simulink library "csu_elk_est_landed_kinematics_lib"  (R2015b)
settings: Solver=ode45  StartTime=0.0  StopTime=10.0  RelTol=1e-3
values from neighbouring files (symbols this model uses):
  elk_body_base_to_origin = 0.25    [csu_elk_est_landed_kinematics_init.m]
undefined symbols (not defined in the file or in its folder): kfl_central_body_radius
libraries: util_common_lib x8, simulink x2, util_info_lib x2
settings Model: Creator=escrane  LastModifiedBy=Mark Agbayani
settings DataIOCC: SaveFormat=Array
settings DebuggingCC: UnderspecifiedInitializationDetection=Classic  MergeDetectMultiDrivingBlocksExec=none  SolverPrmCheckMsg=warning  StateNameClashWarn=warning
settings HardwareCC: ProdBitPerPointer=32  ProdLargestAtomicFloat=None  ProdIntDivRoundTo=Undefined  ProdEndianess=Unspecified  ProdWordSize=32  ProdHWDeviceType=32-bit Generic
settings GRTTargetCC: GeneratePreprocessorConditionals=Disable all
settings ConfigComp: CovModelRefEnable=Off  CovSFcnEnable=off

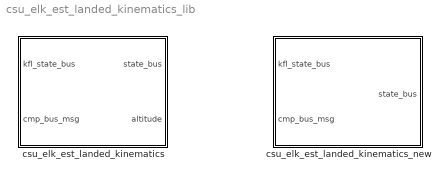
== system csu_elk_est_landed_kinematics_lib ==
  csu_elk_est_landed_kinematics : Subsystem
  csu_elk_est_landed_kinematics_new : Subsystem

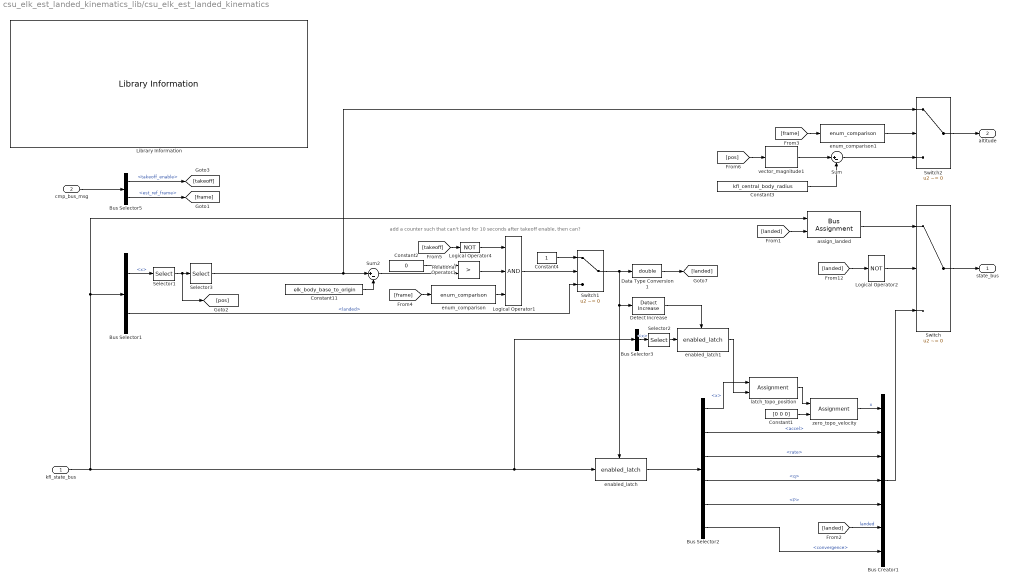
== system csu_elk_est_landed_kinematics_lib/csu_elk_est_landed_kinematics ==
  note: add a counter such that can't land for 10 seconds after takeoff enable, then can?
  kfl_state_bus : Inport
  cmp_bus_msg : Inport  Port=2
  Bus Creator1 : BusCreator  Inputs=7
  Bus Selector1 : BusSelector  OutputSignals=x,landed
  Bus Selector2 : BusSelector  OutputSignals=x,accel,rate,q,P,convergence
  Bus Selector3 : BusSelector  OutputSignals=x
  Bus Selector5 : BusSelector  OutputSignals=takeoff_enable,est_ref_frame
  Constant1 : Constant  Value=[0 0 0]
  Constant11 : Constant  Value=elk_body_base_to_origin  VectorParams1D=off
  Constant2 : Constant  Value=0
  Constant3 : Constant  Value=kfl_central_body_radius  VectorParams1D=off
  Constant4 : Constant
  Data Type Conversion1 : DataTypeConversion  OutDataTypeStr=double
  Detect Increase : simulink/Logic and Bit Operations/Detect Increase  vinit=0  InputProcessing=Inherited  OutDataTypeStr=boolean
  Library Information : util_info_lib/Library Information  owner='escrane'
  Logical Operator1 : Logic  Inputs=3  AllPortsSameDT=off  OutDataTypeStr=boolean
  Logical Operator2 : Logic  Operator=NOT  AllPortsSameDT=off  OutDataTypeStr=boolean
  Logical Operator4 : Logic  Operator=NOT  AllPortsSameDT=off  OutDataTypeStr=boolean
  Relational Operator1 : RelationalOperator  Operator=>  OutDataTypeStr=boolean
  Selector1 : Selector  InputPortWidth=kfl_n_state  IndexOptions=Index vector (dialog)  Indices=kfl_pos_index  OutputSizes=1
  Selector2 : Selector  InputPortWidth=kfl_n_state  IndexOptions=Index vector (dialog)  Indices=kfl_pos_index  OutputSizes=1
  Selector3 : Selector  InputPortWidth=3  IndexOptions=Index vector (dialog)  Indices=[3]  OutputSizes=1
  Sum : Sum  Inputs=|+-
  Sum2 : Sum  Inputs=|+-
  Switch : Switch  Criteria=u2 ~= 0
  Switch1 : Switch  Criteria=u2 ~= 0
  Switch2 : Switch  Criteria=u2 ~= 0
  assign_landed : BusAssignment  AssignedSignals=landed
  enabled_latch : util_common_lib/enabled_latch  initial_output=0
  enabled_latch1 : util_common_lib/enabled_latch  initial_output=0
  enum_comparison : util_common_lib/enum_comparison  comparison_type===
  enum_comparison1 : util_common_lib/enum_comparison  comparison_type===
  latch_topo_position : Assignment  IndexOptions=Index vector (dialog)  Indices=kfl_pos_index  OutputSizes=1
  vector_magnitude1 : util_common_lib/vector_magnitude  SystemSampleTime=-1
  zero_topo_velocity : Assignment  IndexOptions=Index vector (dialog)  Indices=kfl_vel_index  OutputSizes=1
  state_bus : Outport
  altitude : Outport  Port=2
  wires:
  enabled_latch1/1 -> latch_topo_position/2
  Detect Increase/1 -> enabled_latch1/Enable
  Selector2/1 -> enabled_latch1/1
  Bus Selector3/1 -> Selector2/1  "<x>"
  latch_topo_position/1 -> zero_topo_velocity/1
  Selector3/1 -> Switch2/1, Sum2/1
  Bus Selector2/6 -> Bus Creator1/7  "<convergence>"
  Constant3/1 -> Sum/2
  Sum/1 -> Switch2/3
  vector_magnitude1/1 -> Sum/1
  [pos] -> vector_magnitude1/1
  enum_comparison1/1 -> Switch2/2
  [frame] -> enum_comparison1/1
  Switch2/1 -> altitude/1
  [takeoff] -> Logical Operator4/1
  Logical Operator4/1 -> Logical Operator1/1
  Relational Operator1/1 -> Logical Operator1/2
  enum_comparison/1 -> Logical Operator1/3
  Bus Selector1/2 -> Switch1/3  "<landed>"
  Switch1/1 -> Detect Increase/1, enabled_latch/Enable, Data Type Conversion1/1
  Constant4/1 -> Switch1/1
  Logical Operator1/1 -> Switch1/2
  Data Type Conversion1/1 -> [landed]
  [landed] -> assign_landed/2
  assign_landed/1 -> Switch/1
  [landed] -> Bus Creator1/6  "landed"
  [landed] -> Logical Operator2/1
  Sum2/1 -> Relational Operator1/2
  Constant2/1 -> Relational Operator1/1
  Bus Creator1/1 -> Switch/3
  kfl_state_bus/1 -> Bus Selector3/1, enabled_latch/1, assign_landed/1, Bus Selector1/1
  Logical Operator2/1 -> Switch/2
  zero_topo_velocity/1 -> Bus Creator1/1  "x"
  Constant1/1 -> zero_topo_velocity/2
  enabled_latch/1 -> Bus Selector2/1
  Bus Selector2/1 -> latch_topo_position/1  "<x>"
  Bus Selector2/5 -> Bus Creator1/5  "<P>"
  Bus Selector2/2 -> Bus Creator1/2  "<accel>"
  Constant11/1 -> Sum2/2
  Switch/1 -> state_bus/1
  Bus Selector2/3 -> Bus Creator1/3  "<rate>"
  Bus Selector2/4 -> Bus Creator1/4  "<q>"
  Selector1/1 -> Selector3/1, [pos]
  Bus Selector1/1 -> Selector1/1  "<x>"
  Bus Selector5/1 -> [takeoff]  "<takeoff_enable>"
  Bus Selector5/2 -> [frame]  "<est_ref_frame>"
  cmp_bus_msg/1 -> Bus Selector5/1
  [frame] -> enum_comparison/1

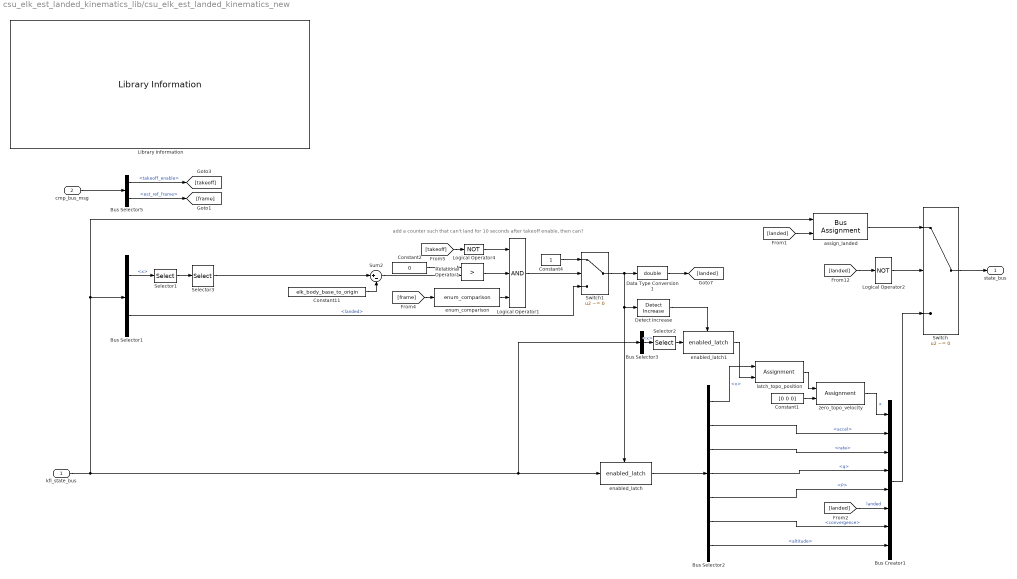
== system csu_elk_est_landed_kinematics_lib/csu_elk_est_landed_kinematics_new ==
  note: add a counter such that can't land for 10 seconds after takeoff enable, then can?
  kfl_state_bus : Inport
  cmp_bus_msg : Inport  Port=2
  Bus Creator1 : BusCreator  Inputs=8
  Bus Selector1 : BusSelector  OutputSignals=x,landed
  Bus Selector2 : BusSelector  OutputSignals=x,accel,rate,q,P,convergence,altitude
  Bus Selector3 : BusSelector  OutputSignals=x
  Bus Selector5 : BusSelector  OutputSignals=takeoff_enable,est_ref_frame
  Constant1 : Constant  Value=[0 0 0]
  Constant11 : Constant  Value=elk_body_base_to_origin  VectorParams1D=off
  Constant2 : Constant  Value=0
  Constant4 : Constant
  Data Type Conversion1 : DataTypeConversion  OutDataTypeStr=double
  Detect Increase : simulink/Logic and Bit Operations/Detect Increase  vinit=0  InputProcessing=Inherited  OutDataTypeStr=boolean
  Library Information : util_info_lib/Library Information  owner='escrane'
  Logical Operator1 : Logic  Inputs=3  AllPortsSameDT=off  OutDataTypeStr=boolean
  Logical Operator2 : Logic  Operator=NOT  AllPortsSameDT=off  OutDataTypeStr=boolean
  Logical Operator4 : Logic  Operator=NOT  AllPortsSameDT=off  OutDataTypeStr=boolean
  Relational Operator1 : RelationalOperator  Operator=>  OutDataTypeStr=boolean
  Selector1 : Selector  InputPortWidth=kfl_n_state  IndexOptions=Index vector (dialog)  Indices=kfl_pos_index  OutputSizes=1
  Selector2 : Selector  InputPortWidth=kfl_n_state  IndexOptions=Index vector (dialog)  Indices=kfl_pos_index  OutputSizes=1
  Selector3 : Selector  InputPortWidth=3  IndexOptions=Index vector (dialog)  Indices=[3]  OutputSizes=1
  Sum2 : Sum  Inputs=|+-
  Switch : Switch  Criteria=u2 ~= 0
  Switch1 : Switch  Criteria=u2 ~= 0
  assign_landed : BusAssignment  AssignedSignals=landed
  enabled_latch : util_common_lib/enabled_latch  initial_output=0
  enabled_latch1 : util_common_lib/enabled_latch  initial_output=0
  enum_comparison : util_common_lib/enum_comparison  comparison_type===
  latch_topo_position : Assignment  IndexOptions=Index vector (dialog)  Indices=kfl_pos_index  OutputSizes=1
  zero_topo_velocity : Assignment  IndexOptions=Index vector (dialog)  Indices=kfl_vel_index  OutputSizes=1
  state_bus : Outport
  wires:
  Bus Selector2/7 -> Bus Creator1/8  "<altitude>"
  enabled_latch1/1 -> latch_topo_position/2
  Detect Increase/1 -> enabled_latch1/Enable
  Selector2/1 -> enabled_latch1/1
  Bus Selector3/1 -> Selector2/1  "<x>"
  latch_topo_position/1 -> zero_topo_velocity/1
  Selector3/1 -> Sum2/1
  Bus Selector2/6 -> Bus Creator1/7  "<convergence>"
  [takeoff] -> Logical Operator4/1
  Logical Operator4/1 -> Logical Operator1/1
  Relational Operator1/1 -> Logical Operator1/2
  enum_comparison/1 -> Logical Operator1/3
  Bus Selector1/2 -> Switch1/3  "<landed>"
  Switch1/1 -> Detect Increase/1, enabled_latch/Enable, Data Type Conversion1/1
  Constant4/1 -> Switch1/1
  Logical Operator1/1 -> Switch1/2
  Data Type Conversion1/1 -> [landed]
  [landed] -> assign_landed/2
  assign_landed/1 -> Switch/1
  [landed] -> Bus Creator1/6  "landed"
  [landed] -> Logical Operator2/1
  Sum2/1 -> Relational Operator1/2
  Constant2/1 -> Relational Operator1/1
  Bus Creator1/1 -> Switch/3
  kfl_state_bus/1 -> Bus Selector3/1, enabled_latch/1, assign_landed/1, Bus Selector1/1
  Logical Operator2/1 -> Switch/2
  zero_topo_velocity/1 -> Bus Creator1/1  "x"
  Constant1/1 -> zero_topo_velocity/2
  enabled_latch/1 -> Bus Selector2/1
  Bus Selector2/1 -> latch_topo_position/1  "<x>"
  Bus Selector2/5 -> Bus Creator1/5  "<P>"
  Bus Selector2/2 -> Bus Creator1/2  "<accel>"
  Constant11/1 -> Sum2/2
  Switch/1 -> state_bus/1
  Bus Selector2/3 -> Bus Creator1/3  "<rate>"
  Bus Selector2/4 -> Bus Creator1/4  "<q>"
  Selector1/1 -> Selector3/1
  Bus Selector1/1 -> Selector1/1  "<x>"
  Bus Selector5/1 -> [takeoff]  "<takeoff_enable>"
  Bus Selector5/2 -> [frame]  "<est_ref_frame>"
  cmp_bus_msg/1 -> Bus Selector5/1
  [frame] -> enum_comparison/1
